simulink model "product_elementwise_test"  (Simulink 9.0)
settings: Solver=FixedStepDiscrete  StartTime=0.0  StopTime=10.0  FixedStep=1.000000  RelTol=1e-3  EnableMultiTasking=on
settings Model: SuppressorTable=22 serialization::archive 11 0 6 0 0 0 0 0  Creator=arnaud  LastModifiedBy=hbourbou
settings DataIOCC: LimitDataPoints=on  SaveFormat=Structure  SignalLoggingSaveFormat=ModelDataLogs
settings OptimizationCC: ExpressionDepthLimit=2147483647
settings DebuggingCC: SolverPrmCheckMsg=warning  FcnCallInpInsideContextMsg=warning  StateNameClashWarn=warning
settings GRTTargetCC: GeneratePreprocessorConditionals=Disable all  CombineOutputUpdateFcns=off  GRTInterface=on
settings ConfigComp: CovSFcnEnable=off

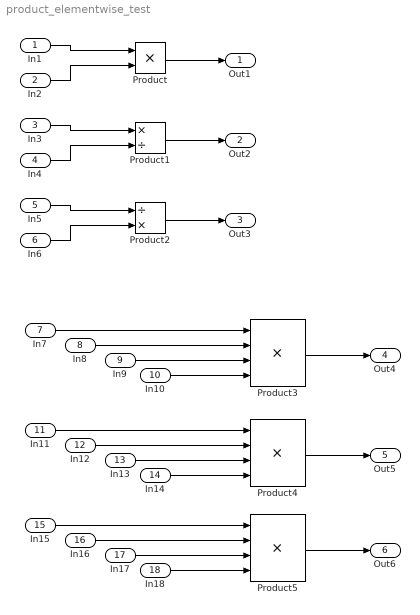
== system product_elementwise_test ==
  In1 : Inport
  In2 : Inport  Port=2
  In3 : Inport  Port=3  PortDimensions=[2]
  In4 : Inport  Port=4  PortDimensions=[2]
  In5 : Inport  Port=5  PortDimensions=[2 2]
  In6 : Inport  Port=6  PortDimensions=[2 2]
  In7 : Inport  Port=7
  In8 : Inport  Port=8
  In9 : Inport  Port=9
  In10 : Inport  Port=10
  In11 : Inport  Port=11  PortDimensions=2
  In12 : Inport  Port=12  PortDimensions=2
  In13 : Inport  Port=13  PortDimensions=2
  In14 : Inport  Port=14  PortDimensions=2
  In15 : Inport  Port=15  PortDimensions=[2 3]
  In16 : Inport  Port=16  PortDimensions=[2 3]
  In17 : Inport  Port=17  PortDimensions=[2 3]
  In18 : Inport  Port=18  PortDimensions=[2 3]
  Product : Product  RndMeth=Zero
  Product1 : Product  Inputs=*/  RndMeth=Zero
  Product2 : Product  Inputs=/*  RndMeth=Zero
  Product3 : Product  Inputs=4  RndMeth=Zero
  Product4 : Product  Inputs=4  RndMeth=Zero
  Product5 : Product  Inputs=4  RndMeth=Zero
  Out1 : Outport
  Out2 : Outport  Port=2
  Out3 : Outport  Port=3
  Out4 : Outport  Port=4
  Out5 : Outport  Port=5
  Out6 : Outport  Port=6
  wires:
  In1/1 -> Product/1
  In2/1 -> Product/2
  Product/1 -> Out1/1
  In3/1 -> Product1/1
  In4/1 -> Product1/2
  Product1/1 -> Out2/1
  In5/1 -> Product2/1
  In6/1 -> Product2/2
  Product2/1 -> Out3/1
  In7/1 -> Product3/1
  In8/1 -> Product3/2
  Product3/1 -> Out4/1
  In9/1 -> Product3/3
  In10/1 -> Product3/4
  In11/1 -> Product4/1
  In12/1 -> Product4/2
  Product4/1 -> Out5/1
  In13/1 -> Product4/3
  In14/1 -> Product4/4
  In15/1 -> Product5/1
  In16/1 -> Product5/2
  Product5/1 -> Out6/1
  In17/1 -> Product5/3
  In18/1 -> Product5/4
